simulink model "subsystem6"  (R2020a)
settings: Solver=FixedStepAuto  StartTime=0.0  StopTime=10.0  FixedStep=0.2  RelTol=1e-3
settings Model: Creator=vijay  LastModifiedBy=Vinayak
settings DataIOCC: SaveOutput=off  SaveTime=off

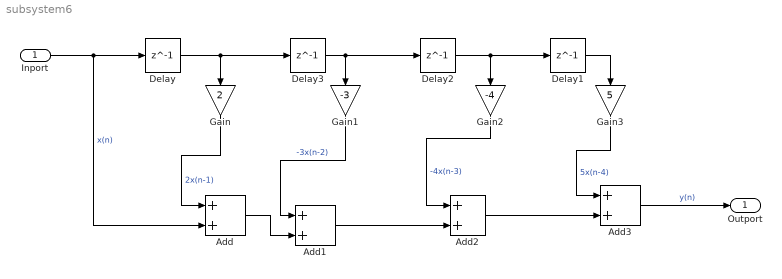
== system subsystem6 ==
  Inport : Inport  OutDataTypeStr=double  PortDimensions=1  SampleTime=[0.20000000000000001,0]
  Add{,1..3} (4 alike) : Sum
  Delay{,1..3} (4 alike) : Delay  DelayLength=1
  Gain : Gain  Gain=2
  Gain1 : Gain  Gain=-3
  Gain2 : Gain  Gain=-4
  Gain3 : Gain  Gain=5
  Outport : Outport  OutDataTypeStr=double  PortDimensions=1  SampleTime=[0.20000000000000001,0]
  wires:
  Add3/1 -> Outport/1  "y(n)"
  Delay2/1 -> Gain2/1, Delay1/1
  Delay/1 -> Delay3/1, Gain/1
  Add2/1 -> Add3/2
  Add/1 -> Add1/2
  Inport/1 -> Delay/1, Add/2  "x(n)"
  Gain3/1 -> Add3/1  "5x(n-4)"
  Add1/1 -> Add2/2
  Gain2/1 -> Add2/1  "-4x(n-3)"
  Gain/1 -> Add/1  "2x(n-1)"
  Delay1/1 -> Gain3/1
  Delay3/1 -> Gain1/1, Delay2/1
  Gain1/1 -> Add1/1  "-3x(n-2)"
